simulink model "Model_DiscreteSignal"  (R2023a)
settings: Solver=ode23t  StartTime=0.0  StopTime=10  MaxStep=0.1  RelTol=1e-4
values from neighbouring files (symbols this model uses):
  k_l = 30    [params_model.m]
  T_1 = 0.1    [params_model.m]
  T_2 = 0.1    [params_model.m]
settings Model: Creator=ПК  LastModifiedBy=ПК

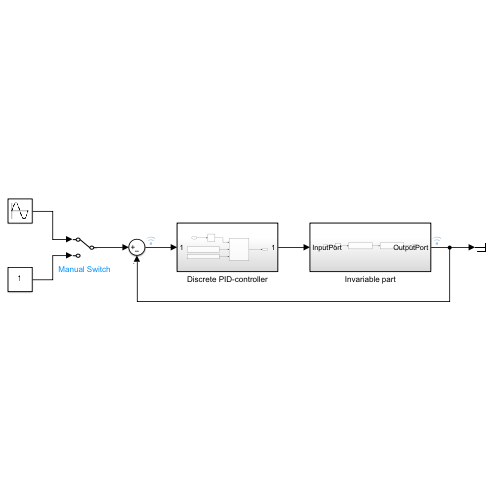
[thumbnail: Simulink's stored preview of the top-level diagram]
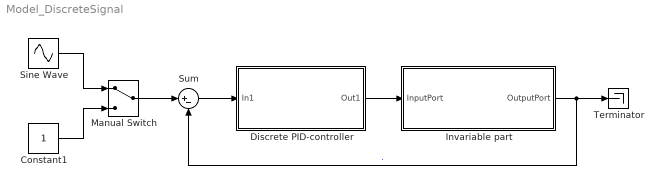
== system Model_DiscreteSignal ==
  Constant1 : Constant
  Discrete PID-controller : Subsystem
  Invariable part : Subsystem
  Manual Switch : ManualSwitch
  Sine Wave : Sin  Amplitude=50  Frequency=0.5  SampleTime=0
  Sum : Sum  Inputs=|+-
  Terminator : Terminator
  wires:
  Sum/1 -> Discrete PID-controller/1(In1)
  Invariable part/1(OutputPort) -> Sum/2, Terminator/1  "."
  Manual Switch/1 -> Sum/1
  Constant1/1 -> Manual Switch/2
  Sine Wave/1 -> Manual Switch/1
  Discrete PID-controller/1(Out1) -> Invariable part/1(InputPort)

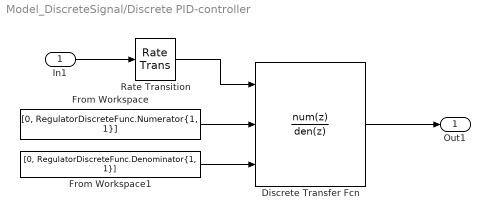
== system Model_DiscreteSignal/Discrete PID-controller ==
  In1 : Inport
  Discrete Transfer Fcn : DiscreteTransferFcn  NumeratorSource=Input port  Numerator="[8.37168601608560\t-16.7038880997959\t8.33224884518259]"  DenominatorSource=Input port  Denominator="[1\t-1.88948213939774\t0.889482139397741]"  a0EqualsOne=on
      settings: InputPortMap=u0,p1,p3
  From Workspace : FromWorkspace  VariableName=[0, RegulatorDiscreteFunc.Numerator{1, 1}]  SampleTime=-1
  From Workspace1 : FromWorkspace  VariableName=[0, RegulatorDiscreteFunc.Denominator{1, 1}]  SampleTime=-1
  Rate Transition : RateTransition  OutPortSampleTime=Ts
  Out1 : Outport
  wires:
  In1/1 -> Rate Transition/1
  From Workspace/1 -> Discrete Transfer Fcn/2
  Discrete Transfer Fcn/1 -> Out1/1
  From Workspace1/1 -> Discrete Transfer Fcn/3
  Rate Transition/1 -> Discrete Transfer Fcn/1

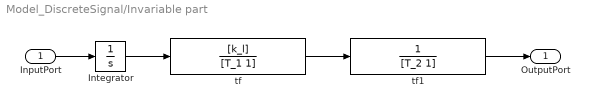
== system Model_DiscreteSignal/Invariable part ==
  InputPort : Inport
  Integrator : Integrator
  tf : TransferFcn  Numerator=[k_l]  Denominator=[T_1 1]
  tf1 : TransferFcn  Denominator=[T_2 1]
  OutputPort : Outport
  wires:
  InputPort/1 -> Integrator/1
  Integrator/1 -> tf/1
  tf/1 -> tf1/1
  tf1/1 -> OutputPort/1
